simulink model "problem1"  (R2020b)
settings: Solver=VariableStepAuto  StartTime=0.0  StopTime=10  RelTol=1e-3
values from neighbouring files (symbols this model uses):
  b = 50    [initalise_values.m]
  k1 = 50    [initalise_values.m]
  k12 = 300    [initalise_values.m]
  m1 = 100    [initalise_values.m]
  m2 = 3    [initalise_values.m]
settings Model: Creator=ARPITA  LastModifiedBy=ARPITA

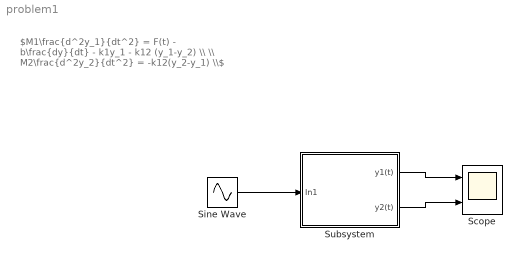
== system problem1 ==
  note: $M1\frac{d^2y_1}{dt^2} = F(t) - b\frac{dy}{dt} - k1y_1 - k12 (y_1-y_2) \\ \\ M2\frac{d^2y_2}{dt^2} = -k12(y_2-y_1) \\$
  Scope : Scope  NumInputPorts=2
  Sine Wave : Sin  Amplitude=2  Frequency=10  SampleTime=0
  Subsystem : Subsystem
  wires:
  Sine Wave/1 -> Subsystem/1(In1)
  Subsystem/1(y1(t)) -> Scope/1
  Subsystem/2(y2(t)) -> Scope/2

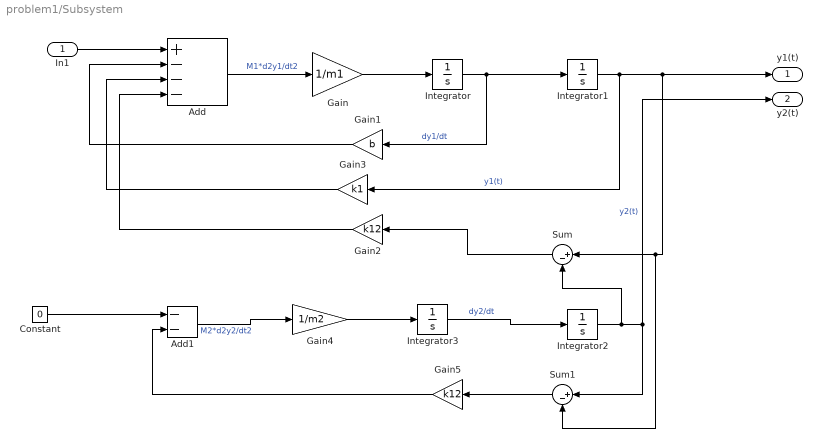
== system problem1/Subsystem ==
  In1 : Inport
  Add : Sum  Inputs=+---
  Add1 : Sum  Inputs=--
  Constant : Constant  Value=0
  Gain : Gain  Gain=1/m1
  Gain1 : Gain  Gain=b
  Gain2 : Gain  Gain=k12
  Gain3 : Gain  Gain=k1
  Gain4 : Gain  Gain=1/m2
  Gain5 : Gain  Gain=k12
  Integrator{,1..3} (4 alike) : Integrator
  Sum : Sum  Inputs=|+-
  Sum1 : Sum  Inputs=|+-
  y1(t) : Outport
  y2(t) : Outport  Port=2
  wires:
  Add1/1 -> Gain4/1  "M2*d2y2/dt2"
  Integrator1/1 -> Gain3/1, y1(t)/1, Sum1/2, Sum/1  "y1(t)"
  Gain5/1 -> Add1/2
  Integrator/1 -> Gain1/1, Integrator1/1  "dy1/dt"
  Integrator3/1 -> Integrator2/1  "dy2/dt"
  Add/1 -> Gain/1  "M1*d2y1/dt2"
  Gain4/1 -> Integrator3/1
  Constant/1 -> Add1/1
  Gain2/1 -> Add/4
  Gain1/1 -> Add/2
  Integrator2/1 -> y2(t)/1, Sum1/1, Sum/2  "y2(t)"
  Gain3/1 -> Add/3
  Sum/1 -> Gain2/1
  Sum1/1 -> Gain5/1
  Gain/1 -> Integrator/1
  In1/1 -> Add/1
